simulink model "model2"  (R2022a)
settings: Solver=ode3  StartTime=0.0  StopTime=2  FixedStep=1e-6  MaxStep=1e-6  RelTol=1e-3
undefined symbols (not defined in the file or in its folder): J, K_1, K_2, K_3, K_4, K_i, K_u, Lm, Lr, Ls, M_nagr, Rs, U_dc, w0_, zp
libraries: nesl_utility x13, fl_lib x12, ee_lib x9, simulink x3
settings Model: Creator=vladi  LastModifiedBy=Family
settings ModelReferenceCC: EnableRefExpFcnMdlSchedulingChecks=off
settings RTWCC: Description=Generic Real-Time Target

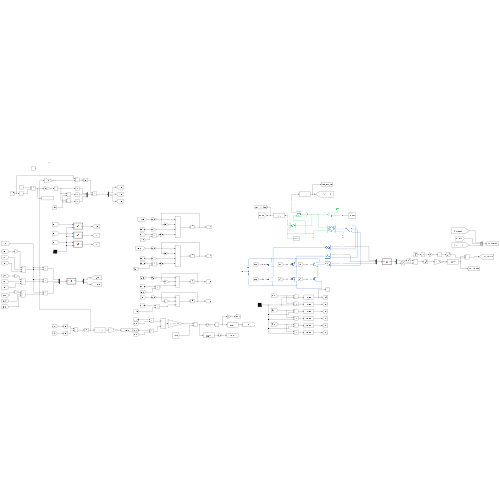
[thumbnail: Simulink's stored preview of the top-level diagram]
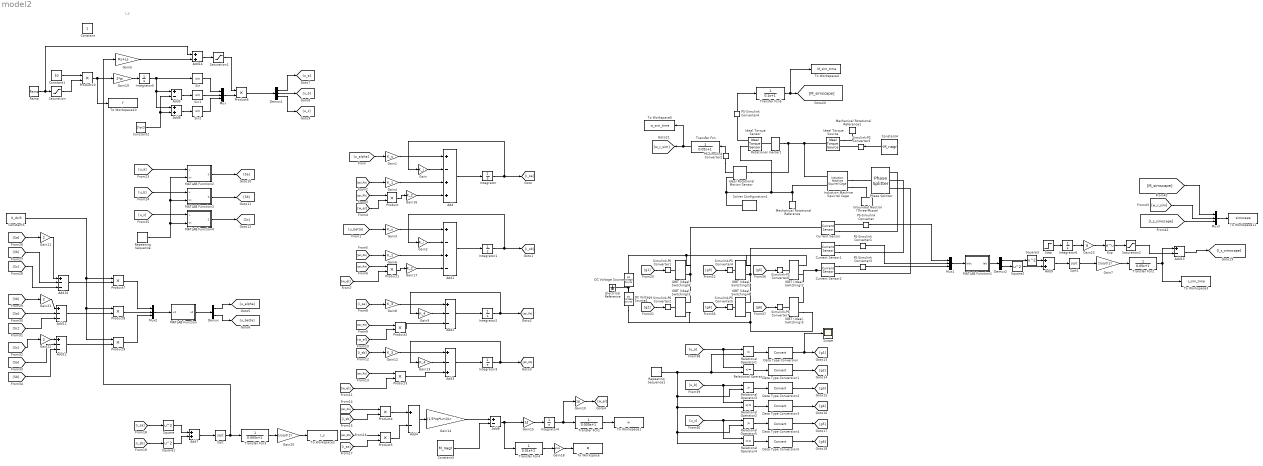
== system model2 ==
  note: I_s
  Add : Sum  Inputs=+-++
  Add1 : Sum  Inputs=+-+-
  Add{2,10..12} (4 alike) : Sum  Inputs=+--
  Add{4..5,8,13} (4 alike) : Sum  Inputs=+-
  Add{6..7,9,14} (4 alike) : Sum
  Add3 : Sum  Inputs=+-+
  Constant : Constant
  Constant1 : Constant  Value=50
  Constant2 : Constant  Value=2*pi/3
  Constant3 : Constant  Value=M_nagr
  Constant4 : Constant  Value=-M_nagr
  Constant5 : Constant  Value=U_dc/3
  Current Sensor : fl_lib/Electrical/Electrical Sensors/Current Sensor
      settings: SourceProductBaseCode=PW,SS,VE
  Current Sensor1 : fl_lib/Electrical/Electrical Sensors/Current Sensor
      settings: SourceProductBaseCode=PW,SS,VE
  Current Sensor2 : fl_lib/Electrical/Electrical Sensors/Current Sensor
      settings: SourceProductBaseCode=PW,SS,VE
  DC Voltage Source : fl_lib/Electrical/Electrical Sources/DC Voltage Source  v0=U_dc/2 V
      settings: SourceProductBaseCode=PW,SS,VE
  DC Voltage Source1 : fl_lib/Electrical/Electrical Sources/DC Voltage Source  v0=U_dc/2 V
      settings: SourceProductBaseCode=PW,SS,VE
  Data Type Conversion{,1..5} (6 alike) : DataTypeConversion  SaturateOnIntegerOverflow=off  RndMeth=Floor
  Demux : Demux  Outputs=2
  Demux1 : Demux  Outputs=3
  Demux2 : Demux  Outputs=2
  Electrical Reference : fl_lib/Electrical/Electrical Elements/Electrical Reference
      settings: SourceProductBaseCode=PW,SS,VE
  Exp : Math
  Gain : Gain  Gain=K_i
  Gain1 : Gain  Gain=K_u
  Gain10 : Gain  Gain=zp
  Gain11 : Gain  Gain=2
  Gain12 : Gain  Gain=K_3
  Gain13 : Gain  Gain=K_4
  Gain14 : Gain  Gain=(1.5*zp*Lm)/Lr
  Gain15 : Gain  Gain=1/J
  Gain16 : Gain  Gain=K_2
  Gain17 : Gain  Gain=K_2
  Gain18 : Gain  Gain=1/1.5
  Gain19 : Gain  Gain=2*pi
  Gain2 : Gain  Gain=K_i
  Gain20 : Gain  Gain=1/sqrt(2)
  Gain21 : Gain  Gain=2
  Gain22 : Gain  Gain=2
  Gain23 : Gain  Gain=8
  Gain3 : Gain  Gain=K_u
  Gain4 : Gain  Gain=K_1
  Gain5 : Gain  Gain=Rs+Ls
  Gain6 : Gain  Gain=K_1
  Gain7 : Gain  Gain=1/sqrt(2)
  Gain8 : Gain  Gain=K_3
  Gain9 : Gain  Gain=K_4
  Grounded Neutral (Three-Phase) : ee_lib/Connectors & References/Grounded Neutral (Three-Phase)
      settings: SourceProductBaseCode=PS
  IGBT (Ideal, Switching){1..6} (6 alike) : ee_lib/Semiconductors & Converters/IGBT (Ideal, Switching)  Vf=0.8 V  Ron=0.001 Ohm  Goff=1e-5 1/Ohm  Vth=.5 V  diode_param=ee.enum.converters.protectiondiode.none  diode_Vf=0.8 V  diode_Ron=0.001 Ohm  diode_Goff=1e-5 1/Ohm  diode_C=50e-9 F  diode_iRM=-235 A  diode_iF=300 A  diode_idot=-50 A/us  diode_trr_param=ee.enum.converters.diodeReverseParam.trr_factor  diode_trr_factor=3  diode_trr=15 us  diode_Qrr=1500 s*uA  thermal_loss_option=ee.enum.converters.thermalLossOption.constantvalues  Von_data=[0, .1, .6, .8, 1, 1.3, 1.6, 2, 2.4; 0, .1, .7, 1, 1.2, 1.5, 1.9, 2.4, 2.8] V  Tj=[298.15, 398.15] K  Iout_data=[0, .1, 1, 5, 10, 20, 40, 70, 100] A  Eon_data=[0, .0024, .024, .12, .2, .48, 1.04, 2.16, 3.24; 0, .003, .03, .15, .25, .6, 1.3, 2.7, 4.05] * 1e-3 J  Eoff_data=[0, .0007, .0066, .033, .066, .17, .33, .83, 1.5; 0, .001, .01, .05, .1, .25, .5, 1.2, 2.2] * 1e-3 J  Tj_loss=[298.15, 398.15] K  Iout_data_loss=[0, .1, 1, 5, 10, 20, 40, 70, 100] A  Eon_scalar=22.86e-3 J  Eoff_scalar=17.14e-3 J  Voff=300 V  Iout_scalar=600 A  diodeModelType=ee.enum.converters.diodeModelType.pwl  diodeTableType=ee.enum.diode.tableType.IfMat  diode_IfMat=[.07, .12, .19, 1.75, 4.24, 7.32, 11.2; .16, .3, .72, 2.14, 4.02, 6.35, 9.12] A  diode_VfMat=[.9, 1.15, 1.25, 1.5, 1.75, 2.17, 2.6, 2.85; .58, .68, .75, 1.1, 1.38, 1.77, 2.27, 2.7] V  diode_TjVec=[25, 125] degC  diode_VfVec=[.5, .7, .9, 1.3, 1.7, 2.1, 2.5] V  diode_IfVec=[.1, .2, .5, 1, 2, 4, 7, 10] A  diode_Vr=-600 V  diode_Ls=150 nH  diode_Erec=0.03 J  thermal_network_parameterization=ee.enum.thermalNetworkTopology.external  Rth=[.08, .5] K/W  Rth_Cauer=[.08, .1, .5] K/W  Rth_Foster=[.08, .14, .22, .16] K/W  thermal_mass_parameterization=ee.enum.thermalNetwork.timeconstant  thermal_mass=[.01, .5] J/K  thermal_mass_Cauer=[.01, .1, .5] J/K  thermal_mass_Foster=[.001, .005, .05, .5] J/K  thermal_time_constant=[.001, .2] s  thermal_time_constant_Cauer=[.001, .1, .2] s  thermal_time_constant_Foster=[7e-05, .0007, .01, .08] s  thermal_mass_initial_temperatures=[25, 25] degC  thermal_mass_initial_temperatures_Cauer=[25, 25, 25] degC  junction_thermal_mass=0.01 J/K  steadyState_Foster=simscape.enum.onoff.on  Tvec_initial_Foster=[25, 25, 25, 25] degC  no_thermal_network=0  junction_temperature_specify=off  junction_temperature_priority=None  junction_temperature=25 degC  junction_temperature_nominal_specify=off  junction_temperature_nominal_unit=degC  junction_temperature_nominal_value=1  vT_specify=off  vT_priority=None  vT=0 V  vT_nominal_specify=off  vT_nominal_unit=V  vT_nominal_value=1  Qj_specify=off  Qj_priority=None  Qj=0 W  Qj_nominal_specify=off  Qj_nominal_unit=W  Qj_nominal_value=1
  Ideal Rotational Motion Sensor : fl_lib/Mechanical/Mechanical Sensors/Ideal Rotational Motion Sensor  wrap_angle=false  offset=0 rad
      settings: SourceProductBaseCode=PW,SS,VE
  Ideal Torque Sensor : fl_lib/Mechanical/Mechanical Sensors/Ideal Torque Sensor
      settings: SourceProductBaseCode=PW,SS,VE
  Ideal Torque Source : fl_lib/Mechanical/Mechanical Sources/Ideal Torque Source
      settings: SourceProductBaseCode=PW,SS,VE
  Induction Machine Squirrel Cage : ee_lib/Electromechanical/Asynchronous/Induction Machine Squirrel Cage  port_option=ee.enum.threePhasePort.composite  SRated=0.75 kW  VRated=220 V  FRated=50 Hz  nPolePairs=3  param_unit=ee.enum.unit.si  squirrel_cage=ee.enum.squirrelcage.Single  zero_sequence=ee.enum.park.zerosequence.include  initialization_option=ee.enum.asm.initialization.fluxvariables  Rs=Rs Ohm  Xls=Ls*w0_ Ohm  pu_Rs=0.0258  pu_Lls=0.0413  Rrd=Rr Ohm  Xlrd=Lr*w0_ Ohm  pu_Rrd=0.0145  pu_Llrd=0.0424  Rrd1=0.28 Ohm  Xlrd1=0.82 Ohm  Rrd2=0.28 Ohm  Xlrd2=0.82 Ohm  pu_Rrd1=0.0290  pu_Llrd1=0.0848  pu_Rrd2=0.0290  pu_Llrd2=0.0848  Xm=Lm*w0_ Ohm  pu_Lm=1.7562  X0=0.4 Ohm  pu_L0=0.0413  saturation_option=ee.enum.saturation.exclude  saturation_i=[0, 4, 9, 18, 25, 34, 50, 68, 95, 120] A  saturation_v=[0, 88, 154, 198, 220, 242, 264, 286, 308, 327] V  pu_saturation_i=[0, .176, .396, .792, 1.1, 1.496, 2.2, 2.992, 4.18, 5.28]  pu_saturation_v=[0, .4, .7, .9, 1, 1.1, 1.2, 1.3, 1.4, 1.4864]  connection_option=ee.enum.Connection.delta  angular_position_specify=off  angular_position_priority=None  angular_position=0 deg  angular_position_nominal_specify=off  angular_position_nominal_unit=deg  angular_position_nominal_value=1  pu_psids_specify=off  pu_psids_priority=None  pu_psids=0  pu_psids_nominal_specify=off  pu_psids_nominal_unit=1  pu_psids_nominal_value=1  pu_psiqs_specify=off  pu_psiqs_priority=None  pu_psiqs=0  pu_psiqs_nominal_specify=off  pu_psiqs_nominal_unit=1  pu_psiqs_nominal_value=1  pu_psi0s_specify=off  pu_psi0s_priority=None  pu_psi0s=0  pu_psi0s_nominal_specify=off  pu_psi0s_nominal_unit=1  pu_psi0s_nominal_value=1  pu_psidr_specify=off  pu_psidr_priority=None  pu_psidr=0  pu_psidr_nominal_specify=off  pu_psidr_nominal_unit=1  pu_psidr_nominal_value=1  pu_psiqr_specify=off  pu_psiqr_priority=None  pu_psiqr=0  pu_psiqr_nominal_specify=off  pu_psiqr_nominal_unit=1  pu_psiqr_nominal_value=1  pu_psidr1_specify=off  pu_psidr1_priority=None  pu_psidr1=0  pu_psidr1_nominal_specify=off  pu_psidr1_nominal_unit=1  pu_psidr1_nominal_value=1  pu_psiqr1_specify=off  pu_psiqr1_priority=None  pu_psiqr1=0  pu_psiqr1_nominal_specify=off  pu_psiqr1_nominal_unit=1  pu_psiqr1_nominal_value=1  pu_psidr2_specify=off  pu_psidr2_priority=None  pu_psidr2=0  pu_psidr2_nominal_specify=off  pu_psidr2_nominal_unit=1  pu_psidr2_nominal_value=1  pu_psiqr2_specify=off  pu_psiqr2_priority=None  pu_psiqr2=0  pu_psiqr2_nominal_specify=off  pu_psiqr2_nominal_unit=1  pu_psiqr2_nominal_value=1  psids_specify=off  psids_priority=None  psids=0 Wb  psids_nominal_specify=off  psids_nominal_unit=Wb  psids_nominal_value=1  psiqs_specify=off  psiqs_priority=None  psiqs=0 Wb  psiqs_nominal_specify=off  psiqs_nominal_unit=Wb  psiqs_nominal_value=1  psi0s_specify=off  psi0s_priority=None  psi0s=0 Wb  psi0s_nominal_specify=off  psi0s_nominal_unit=Wb  psi0s_nominal_value=1  psidr_specify=off  psidr_priority=None  psidr=0 Wb  psidr_nominal_specify=off  psidr_nominal_unit=Wb  psidr_nominal_value=1  psiqr_specify=off  psiqr_priority=None  psiqr=0 Wb  psiqr_nominal_specify=off  psiqr_nominal_unit=Wb  psiqr_nominal_value=1  psidr1_specify=off  psidr1_priority=None  psidr1=0 Wb  psidr1_nominal_specify=off  psidr1_nominal_unit=Wb  psidr1_nominal_value=1  psiqr1_specify=off  psiqr1_priority=None  psiqr1=0 Wb  psiqr1_nominal_specify=off  psiqr1_nominal_unit=Wb  psiqr1_nominal_value=1  psidr2_specify=off  psidr2_priority=None  psidr2=0 Wb  psidr2_nominal_specify=off  psidr2_nominal_unit=Wb  psidr2_nominal_value=1  psiqr2_specify=off  psiqr2_priority=None  psiqr2=0 Wb  psiqr2_nominal_specify=off  psiqr2_nominal_unit=Wb  psiqr2_nominal_value=1  slip_specify=off  slip_priority=None  slip=0  slip_nominal_specify=off  slip_nominal_unit=1  slip_nominal_value=1  real_power_generated_specify=off  real_power_generated_priority=None  real_power_generated=0 W  real_power_generated_nominal_specify=off  real_power_generated_nominal_unit=W  real_power_generated_nominal_value=1  mechanical_power_consumed_specify=off  mechanical_power_consumed_priority=None  mechanical_power_consumed=0 W  mechanical_power_consumed_nominal_specify=off  mechanical_power_consumed_nominal_unit=W  mechanical_power_consumed_nominal_value=1  Tmeas=298.15 K  alpha=3.93e-3 1/K  alpha_cage=4.4e-3 1/K  stator_thermal_mass=100 J/K  rotor_thermal_mass=200 J/K  temperatureA_specify=off  temperatureA_priority=High  temperatureA=25 degC  temperatureA_nominal_specify=off  temperatureA_nominal_unit=degC  temperatureA_nominal_value=1  temperatureB_specify=off  temperatureB_priority=High  temperatureB=25 degC  temperatureB_nominal_specify=off  temperatureB_nominal_unit=degC  temperatureB_nominal_value=1  temperatureC_specify=off  temperatureC_priority=High  temperatureC=25 degC  temperatureC_nominal_specify=off  temperatureC_nominal_unit=degC  temperatureC_nominal_value=1  temperatureR_specify=off  temperatureR_priority=High  temperatureR=25 degC  temperatureR_nominal_specify=off  temperatureR_nominal_unit=degC  temperatureR_nominal_value=1
      settings: SourceProductBaseCode=PS  LogSimulationData=on  InternalSimscapePortConfiguration="{\"Bottom\":[],\"Left\":[{\"id\":\"R\",\"label\":\"R\",\"type\":\"foundation.mechanical.rotational.rotational\"},{\"id\":\"C\",\"label\":\"C\",\"type\":\"foundation.mechanical.rotational.rotational\"}],\"Right\":[{\"id\":\"pu_output\",\"label\":\"pu\",\"type\":\"output\"},{\"id\":\"N1\",\"label\":\"~1\",\"type\":\"foundation.electrical.three_phase\"},{\"id\":\"N2\",\"label\":\"~2\",\"type\":\"foundation.electrical.three_phase\"}],\"Top\":[]}"
  Integrator{,1..6} (7 alike) : Integrator
  MATLAB Function : MATLAB Function  TreatAsAtomicUnit=on  SystemSampleTime=1e-6
  MATLAB Function1 : MATLAB Function  TreatAsAtomicUnit=on  SystemSampleTime=1e-6
  MATLAB Function2 : MATLAB Function  TreatAsAtomicUnit=on  SystemSampleTime=1e-6
  MATLAB Function3 : MATLAB Function  TreatAsAtomicUnit=on  SystemSampleTime=1e-6
  MATLAB Function4 : MATLAB Function  TreatAsAtomicUnit=on  SystemSampleTime=1e-6
  Mechanical Rotational Reference : fl_lib/Mechanical/Rotational Elements/Mechanical Rotational Reference
      settings: SourceProductBaseCode=PW,SS,VE
  Mechanical Rotational Reference1 : fl_lib/Mechanical/Rotational Elements/Mechanical Rotational Reference
      settings: SourceProductBaseCode=PW,SS,VE
  Mux{,1..3} (4 alike) : Mux  Inputs=3
  PS-Simulink Converter{,1..4} (5 alike) : nesl_utility/PS-Simulink Converter  PhysicalDomain=network_engine_domain  SubClassName=ps_output  LeftPortType=input  RightPortType=output  PseudoPeriodic=off  Frequencies=[]  VectorFormat=1-D array  Unit=inherit  AffineConversion=off
      settings: SourceProductBaseCode=SS,PW,VE
  Phase Splitter : ee_lib/Connectors & References/Phase Splitter
      settings: SourceProductBaseCode=PS
  Product{,1..10} (11 alike) : Product
  Ramp : simulink/Sources/Ramp  slope=1.2  start=0  InitialOutput=0
  Relational Operator : RelationalOperator  Operator=<=  OutDataTypeStr=boolean  RndMeth=Simplest  InputSameDT=off
  Relational Operator1 : RelationalOperator  Operator=>  OutDataTypeStr=boolean  RndMeth=Simplest  InputSameDT=off
  Relational Operator2 : RelationalOperator  Operator=<=  OutDataTypeStr=boolean  RndMeth=Simplest  InputSameDT=off
  Relational Operator3 : RelationalOperator  Operator=>  OutDataTypeStr=boolean  RndMeth=Simplest  InputSameDT=off
  Relational Operator4 : RelationalOperator  Operator=<=  OutDataTypeStr=boolean  RndMeth=Simplest  InputSameDT=off
  Relational Operator5 : RelationalOperator  Operator=>  OutDataTypeStr=boolean  RndMeth=Simplest  InputSameDT=off
  Repeating Sequence : simulink/Sources/Repeating Sequence  rep_seq_t=[0 1/10000 1/5000]  rep_seq_y=[-1 1 -1]
  Repeating Sequence1 : simulink/Sources/Repeating Sequence  rep_seq_t=[0 1/10000 1/5000]  rep_seq_y=[-1 1 -1]
  Rotational Inerter1 : fl_lib/Mechanical/Rotational Elements/Rotational Inerter  B=J kg*m^2  w_specify=off  w_priority=High  w=0 rad/s  w_nominal_specify=off  w_nominal_unit=rad/s  w_nominal_value=1  t_specify=off  t_priority=None  t=0 N*m  t_nominal_specify=off  t_nominal_unit=N*m  t_nominal_value=1
      settings: SourceProductBaseCode=PW,SS,VE  InternalSimscapePortConfiguration="{\"Bottom\":[],\"Left\":[{\"id\":\"R\",\"label\":\"R\",\"type\":\"foundation.mechanical.rotational.rotational\"}],\"Right\":[{\"id\":\"C\",\"label\":\"C\",\"type\":\"foundation.mechanical.rotational.rotational\"}],\"Top\":[]}"
  Saturation : Saturate  UpperLimit=1  LowerLimit=0
  Saturation1 : Saturate  UpperLimit=1  LowerLimit=0
  Saturation2 : Saturate  UpperLimit=2.9  LowerLimit=0
  Scope : Scope
  Simulink-PS Converter{1..7} (7 alike) : nesl_utility/Simulink-PS Converter  PhysicalDomain=network_engine_domain  SubClassName=ps_input  LeftPortType=input  RightPortType=output  PseudoPeriodic=off  Frequencies=[]  NoiseDistribution=none  NoiseParameters=[]  Unit=1  AffineConversion=off  FilteringAndDerivatives=provide  SimscapeFilterOrder=1  InputFilterTimeConstant=0.001  UdotUserProvided=0
      settings: SourceProductBaseCode=SS,PW,VE
  Sin : Trigonometry
  Sin1 : Trigonometry
  Sin2 : Trigonometry
  Solver Configuration1 : nesl_utility/Solver Configuration  PhysicalDomain=network_engine_domain  SubClassName=solver  LeftPortType=input  RightPortType=generic  Tones=[]  Harmonics=[]  SimulateNoise=off  Profile=off  UseLocalSampling=off  EnableSwitchedLinearOptims=on  FrequencyDomain=off  UseCCode=off  RelTol=0.001  AbsTol=0.001  MinStep=1e-09  ToWorkspace=off  RevertToSquareIcSolve=off  NumHomotopyIterations=100  PhasorMode=off  PhasorModeNumHarmonics=1  IndexReductionMethod=DerivativeReplacement  DoDC=off  ResidualTolerance=1e-09  UseLocalSolver=on  LocalSolverChoice=NE_TRAPEZOIDAL_ADVANCER  LocalSolverSampleTime=1e-6  DoFixedCost=on  MaxNonlinIter=3  MaxModeIter=2  ComputeImpulses=off  ImpulseIterations=2  LinearAlgebra=auto  LinearAlgebraNumThread=0  EquationFormulation=NE_TIME_EF  DelaysMemoryBudget=1024  AutomaticFiltering=on  FilteringTimeConstant=0.001  PartitionStorageMethod=AS_NEEDED  PartitionMemoryBudget=1024  PartitionMethod=ROBUST
      settings: SourceProductBaseCode=SS,PW,VE
  Sqrt : Sqrt
  Sqrt1 : Sqrt
  Square{,1..3} (4 alike) : Math  Operator=square
  Step : Step  Time=0.1  SampleTime=0
  To Workspace : ToWorkspace  VariableName=M  SaveFormat=Timeseries  SampleTime=-1
  To Workspace1 : ToWorkspace  VariableName=w  SaveFormat=Timeseries  SampleTime=-1
  To Workspace10 : ToWorkspace  VariableName=f  SaveFormat=Timeseries  SampleTime=-1
  To Workspace11 : ToWorkspace  VariableName=simscape  SampleTime=-1
  To Workspace2 : ToWorkspace  VariableName=I_s  SaveFormat=Timeseries  SampleTime=-1
  To Workspace3 : ToWorkspace  VariableName=I_sim_time  SaveFormat=Timeseries  SampleTime=-1
  To Workspace4 : ToWorkspace  VariableName=M_sim_time  SaveFormat=Timeseries  SampleTime=-1
  To Workspace5 : ToWorkspace  VariableName=w_sim_time  SaveFormat=Timeseries  SampleTime=-1
  Transfer Fcn : TransferFcn  Denominator=[0.05 1]
  Transfer Fcn1 : TransferFcn  Denominator=[0.005 1]
  Transfer Fcn2 : TransferFcn  Denominator=[0.05 1]
  Transfer Fcn3 : TransferFcn  Denominator=[0.005 1]
  Transfer Fcn4 : TransferFcn  Denominator=[0.01 1]
  Transfer Fcn5 : TransferFcn  Denominator=[0.1 1]
  wires:
  Add/1 -> Integrator/1
  Gain/1 -> Add/2
  [u_alpha] -> Gain1/1
  Gain1/1 -> Add/1
  Gain3/1 -> Add1/1
  Add1/1 -> Integrator1/1
  [u_betta] -> Gain3/1
  Gain2/1 -> Add1/2
  Integrator/1 -> [i_sa], Gain/1
  Integrator1/1 -> [i_sb], Gain2/1
  Add2/1 -> Integrator2/1
  [psi_Ra] -> Gain4/1
  Gain4/1 -> Add/3
  [w_el] -> Product/2
  [psi_Rb] -> Product/1
  Product/1 -> Gain16/1
  Gain6/1 -> Add1/3
  [psi_Rb] -> Gain6/1
  Product1/1 -> Gain17/1
  [w_el] -> Product1/2
  [psi_Ra] -> Product1/1
  [i_sa] -> Gain8/1
  Gain8/1 -> Add2/1
  Gain9/1 -> Add2/2
  Integrator2/1 -> [psi_Ra], Gain9/1
  [w_el] -> Product2/2
  [psi_Rb] -> Product2/1
  Product2/1 -> Add2/3
  [psi_Ra] -> Product3/1
  [w_el] -> Product3/2
  Gain13/1 -> Add3/2
  Product3/1 -> Add3/3
  Gain12/1 -> Add3/1
  Integrator3/1 -> [psi_Rb], Gain13/1
  [i_sb] -> Gain12/1
  Add3/1 -> Integrator3/1
  Add4/1 -> Gain14/1
  Product4/1 -> Add4/1
  Product5/1 -> Add4/2
  [psi_Ra] -> Product4/1
  [psi_Rb] -> Product5/1
  Gain16/1 -> Add/4
  Gain17/1 -> Add1/4
  Gain19/1 -> Integrator5/1
  Integrator5/1 -> Add6/1, Add5/1, Sin/1
  Constant2/1 -> Add5/2, Add6/2
  Add5/1 -> Sin1/1
  Add6/1 -> Sin2/1
  Sin2/1 -> Mux/3
  Sin1/1 -> Mux/2
  Sin/1 -> Mux/1
  Mux/1 -> Product6/2
  Product6/1 -> Demux1/1
  Demux1/1 -> [u_a]
  Demux1/2 -> [u_b]
  Demux1/3 -> [u_c]
  [i_sa] -> Square/1
  [i_sb] -> Square1/1
  Square/1 -> Add7/1
  Square1/1 -> Add7/2
  Add7/1 -> Sqrt/1
  Sqrt/1 -> Transfer Fcn3/1, Gain5/1
  PS-Simulink Converter/1 -> Mux1/1
  [i_sb] -> Product4/2
  [i_sa] -> Product5/2
  PS-Simulink Converter2/1 -> Transfer Fcn/1
  Add8/1 -> Gain15/1, Transfer Fcn4/1
  Gain14/1 -> Add8/1
  Constant3/1 -> Add8/2
  Constant4/1 -> Simulink-PS Converter3/1
  Sqrt1/1 -> Gain7/1
  PS-Simulink Converter3/1 -> Mux1/3
  PS-Simulink Converter1/1 -> Mux1/2
  MATLAB Function1/1(Iab) -> Demux2/1
  Mux1/1 -> MATLAB Function1/1(Iabc)
  Demux2/2 -> Square2/1
  Square2/1 -> Add9/2
  Square3/1 -> Add9/1
  Demux2/1 -> Square3/1
  Add9/1 -> Sqrt1/1
  Gain15/1 -> Integrator4/1
  Gain10/1 -> [w_el]
  Integrator4/1 -> Transfer Fcn1/1, Gain10/1
  Gain7/1 -> Transfer Fcn2/1
  Ramp/1 -> Add14/1, Saturation/1
  [u_a] -> MATLAB Function2/1(u)
  Repeating Sequence/1 -> MATLAB Function4/2(tri), MATLAB Function3/2(tri), MATLAB Function2/2(tri)
  [u_c] -> MATLAB Function4/1(u)
  [u_b] -> MATLAB Function3/1(u)
  MATLAB Function2/1(S) -> [Sa]
  MATLAB Function3/1(S) -> [Sb]
  MATLAB Function4/1(S) -> [Sc]
  MATLAB Function/1(u2) -> Demux/1
  Demux/1 -> [u_alpha]
  Demux/2 -> [u_betta]
  Mux2/1 -> MATLAB Function/1(u3)
  Product7/1 -> Mux2/1
  Constant5/1 -> Product7/1, Product8/1, Product9/1
  Product8/1 -> Mux2/2
  Product9/1 -> Mux2/3
  Add12/1 -> Product9/2
  Add11/1 -> Product8/2
  Add10/1 -> Product7/2
  [Sa] -> Gain11/1
  Gain11/1 -> Add10/1
  [Sb] -> Add10/2
  [Sc] -> Add10/3
  [Sa] -> Add11/2
  [Sc] -> Add11/3
  [Sc] -> Gain22/1
  [Sa] -> Add12/2
  [Sb] -> Add12/3
  Gain21/1 -> Add11/1
  [Sb] -> Gain21/1
  Gain22/1 -> Add12/1
  [g1] -> Simulink-PS Converter1/1
  [g2] -> Simulink-PS Converter2/1
  [g3] -> Simulink-PS Converter4/1
  [g4] -> Simulink-PS Converter5/1
  [g5] -> Simulink-PS Converter6/1
  [g6] -> Simulink-PS Converter7/1
  Relational Operator1/1 -> Data Type Conversion/1
  Relational Operator/1 -> Data Type Conversion1/1
  Relational Operator3/1 -> Data Type Conversion2/1
  Relational Operator2/1 -> Data Type Conversion3/1
  Relational Operator5/1 -> Data Type Conversion4/1
  Relational Operator4/1 -> Data Type Conversion5/1
  [u_a] -> Relational Operator/1, Relational Operator1/1
  Repeating Sequence1/1 -> Relational Operator/2, Relational Operator1/2, Relational Operator3/2, Relational Operator2/2, Relational Operator4/2, Relational Operator5/2
  [u_b] -> Relational Operator2/1, Relational Operator3/1
  [u_c] -> Relational Operator4/1, Relational Operator5/1
  Data Type Conversion/1 -> Scope/1, [g1]
  Data Type Conversion1/1 -> [g2]
  Data Type Conversion2/1 -> [g3]
  Data Type Conversion3/1 -> [g4]
  Data Type Conversion4/1 -> [g5]
  Data Type Conversion5/1 -> [g6]
  PS-Simulink Converter4/1 -> Transfer Fcn5/1
  Transfer Fcn/1 -> To Workspace5/1, [w_r_sim]
  Transfer Fcn5/1 -> To Workspace4/1, [M_simscape]
  Mux3/1 -> To Workspace11/1
  Transfer Fcn2/1 -> Add13/1, To Workspace3/1
  [I_s_simscape] -> Mux3/3
  [M_simscape] -> Mux3/1
  [w_r_sim] -> Mux3/2
  Add13/1 -> [I_s_simscape]
  Product10/1 -> To Workspace10/1, Gain19/1
  Constant1/1 -> Product10/1
  Saturation/1 -> Product10/2
  Add14/1 -> Saturation1/1
  Transfer Fcn3/1 -> Gain20/1
  Transfer Fcn4/1 -> Gain18/1
  Saturation1/1 -> Product6/1
  Gain20/1 -> To Workspace2/1
  Transfer Fcn1/1 -> To Workspace1/1
  Gain18/1 -> To Workspace/1
  Integrator6/1 -> Gain23/1
  Gain23/1 -> Exp/1
  Step/1 -> Integrator6/1
  Exp/1 -> Saturation2/1
  Gain5/1 -> Add14/2
  Saturation2/1 -> Add13/2
  connections:
  PS-Simulink Converter/LConn1 -- Current Sensor/RConn1
  Current Sensor/RConn2 -- Phase Splitter/RConn1
  Current Sensor1/RConn2 -- Phase Splitter/RConn2
  Current Sensor2/RConn2 -- Phase Splitter/RConn3
  Induction Machine Squirrel Cage/RConn2 -- Phase Splitter/LConn1
  Induction Machine Squirrel Cage/RConn3 -- Grounded Neutral (Three-Phase)/LConn1
  Rotational Inerter1/LConn1 -- Ideal Rotational Motion Sensor/LConn1 -- Ideal Torque Source/LConn1 -- Induction Machine Squirrel Cage/LConn1
  Ideal Rotational Motion Sensor/RConn1 -- Solver Configuration1/RConn1 -- Ideal Torque Sensor/RConn1 -- Induction Machine Squirrel Cage/LConn2 -- Mechanical Rotational Reference/LConn1
  Ideal Torque Source/RConn2 -- Mechanical Rotational Reference1/LConn1
  Simulink-PS Converter3/RConn1 -- Ideal Torque Source/RConn1
  Current Sensor1/RConn1 -- PS-Simulink Converter1/LConn1
  Current Sensor2/RConn1 -- PS-Simulink Converter3/LConn1
  DC Voltage Source/RConn1 -- DC Voltage Source1/LConn1 -- Electrical Reference/LConn1
  "IGBT (Ideal, Switching)2"/RConn1 -- "IGBT (Ideal, Switching)1"/RConn1 -- "IGBT (Ideal, Switching)6"/RConn1 -- DC Voltage Source/LConn1
  Current Sensor2/LConn1 -- "IGBT (Ideal, Switching)2"/RConn2 -- "IGBT (Ideal, Switching)5"/RConn1
  "IGBT (Ideal, Switching)3"/RConn2 -- DC Voltage Source1/RConn1 -- "IGBT (Ideal, Switching)5"/RConn2 -- "IGBT (Ideal, Switching)4"/RConn2
  Current Sensor/LConn1 -- "IGBT (Ideal, Switching)3"/RConn1 -- "IGBT (Ideal, Switching)6"/RConn2
  Current Sensor1/LConn1 -- "IGBT (Ideal, Switching)4"/RConn1 -- "IGBT (Ideal, Switching)1"/RConn2
  "IGBT (Ideal, Switching)6"/LConn1 -- Simulink-PS Converter1/RConn1
  "IGBT (Ideal, Switching)3"/LConn1 -- Simulink-PS Converter2/RConn1
  "IGBT (Ideal, Switching)1"/LConn1 -- Simulink-PS Converter4/RConn1
  "IGBT (Ideal, Switching)4"/LConn1 -- Simulink-PS Converter5/RConn1
  "IGBT (Ideal, Switching)2"/LConn1 -- Simulink-PS Converter6/RConn1
  "IGBT (Ideal, Switching)5"/LConn1 -- Simulink-PS Converter7/RConn1
  PS-Simulink Converter2/LConn1 -- Ideal Rotational Motion Sensor/RConn2
  Ideal Torque Sensor/RConn2 -- PS-Simulink Converter4/LConn1
  Rotational Inerter1/RConn1 -- Ideal Torque Sensor/LConn1

== matlab function model2/MATLAB Function ==
  data: u3 input; u2 output
function u2 = fcn(u3)
    u2 = [2/3 -(1/3) -(1/3);0 1/sqrt(3) -1/sqrt(3)] * u3;
end

== matlab function model2/MATLAB Function2 ==
  data: u input; S output; tri input
function S = fcn(u, tri)
if u>= tri 
    S = 1;
else
    S=0;
end

== matlab function model2/MATLAB Function3 ==
  data: u input; S output; tri input
function S = fcn(u, tri)
if u>= tri 
    S = 1;
else
    S=0;
end

== matlab function model2/MATLAB Function4 ==
  data: u input; S output; tri input
function S = fcn(u, tri)
if u>= tri 
    S = 1;
else
    S=0;
end

== matlab function model2/MATLAB Function1 ==
  data: Iabc input; Iab output
function Iab = fcn(Iabc)
    Iab = [2/3 -(1/3) -(1/3);0 1/sqrt(3) -1/sqrt(3)] * Iabc;
end
